simulink model "arm_sim_SMC"  (R2013a)
settings: Solver=ode45  StartTime=0.0  StopTime=100  RelTol=1e-3
undefined symbols (not defined in the file or in its folder): arm_ctrl, drawArm
settings Model: Creator=beard  LastModifiedBy=daqing_yi
settings DataIOCC: SignalLoggingSaveFormat=ModelDataLogs
settings OptimizationCC: ExpressionDepthLimit=2147483647  InitFltsAndDblsToZero=on
settings DebuggingCC: MultiTaskDSMMsg=warning  MultiTaskCondExecSysMsg=none  FcnCallInpInsideContextMsg=UseLocalSettings  StrictBusMsg=None
settings RTWCC: IncludeERTFirstTime=on
settings GRTTargetCC: CombineOutputUpdateFcns=off  GRTInterface=on

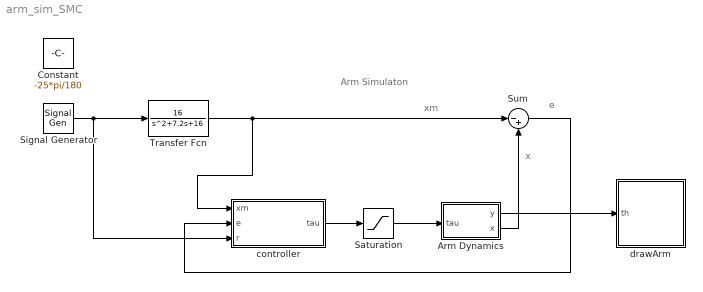
== system arm_sim_SMC ==
  note: x
  note: xm
  note: e
  note: Arm Simulaton
  Arm Dynamics : Subsystem
  Constant : Constant  Value=-25*pi/180
  Saturation : Saturate  UpperLimit=2  LowerLimit=-2
  Signal Generator : SignalGenerator  WaveForm=square  Amplitude=25*pi/180  Frequency=.05
  Sum : Sum  Inputs=|-+
  Transfer Fcn : TransferFcn  Numerator=[16]  Denominator=[1 7.2 16]
  controller : Subsystem
  drawArm : Subsystem
      mask init:
      | % drawing parameters
      | L = 1;
      | w = 0.3;
      mask Display: image(imread('tv.jpg'))
  wires:
  controller/1(tau) -> Saturation/1
  Saturation/1 -> Arm Dynamics/1(tau)
  Arm Dynamics/1(y) -> drawArm/1(th)
  Signal Generator/1 -> controller/3(r), Transfer Fcn/1
  Transfer Fcn/1 -> Sum/1, controller/1(xm)
  Arm Dynamics/2(x) -> Sum/2
  Sum/1 -> controller/2(e)

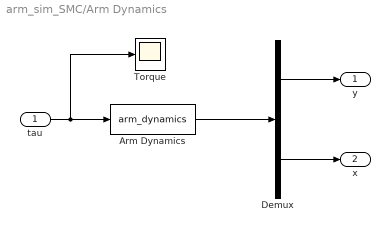
== system arm_sim_SMC/Arm Dynamics ==
  tau : Inport
  Arm Dynamics : S-Function  FunctionName=arm_dynamics  EnableBusSupport=off
  Demux : Demux  Outputs=[1;2]
  Torque : Scope
      settings: TimeRange=100  YMin=-1  YMax=2  SaveName=ScopeData2
  y : Outport
  x : Outport  Port=2
  wires:
  tau/1 -> Arm Dynamics/1, Torque/1
  Arm Dynamics/1 -> Demux/1
  Demux/1 -> y/1
  Demux/2 -> x/1

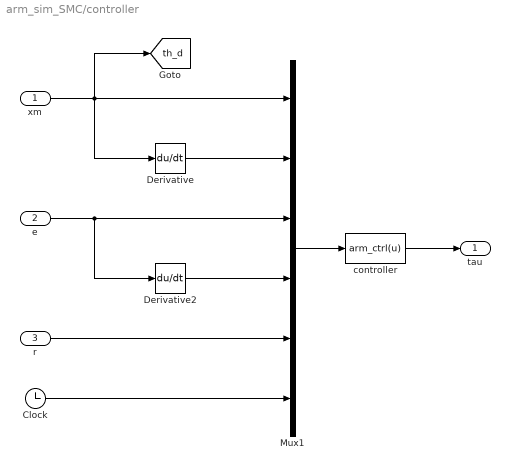
== system arm_sim_SMC/controller ==
  xm : Inport
  e : Inport  Port=2
  r : Inport  Port=3
  Clock : Clock
  Derivative : Derivative
  Derivative2 : Derivative
  Mux1 : Mux  Inputs=6
  controller : MATLABFcn  MATLABFcn=arm_ctrl(u)  OutputDimensions=1  SampleTime=0.01
  tau : Outport
  tag scope: th_d=global
  wires:
  Mux1/1 -> controller/1
  controller/1 -> tau/1
  Clock/1 -> Mux1/6
  xm/1 -> [th_d], Derivative/1, Mux1/1
  Derivative/1 -> Mux1/2
  e/1 -> Mux1/3, Derivative2/1
  Derivative2/1 -> Mux1/4
  r/1 -> Mux1/5

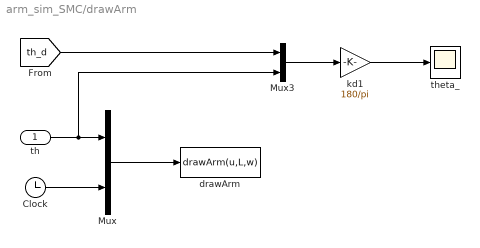
== system arm_sim_SMC/drawArm ==
  th : Inport
  Clock : Clock
  Mux : Mux  Inputs=2
  Mux3 : Mux  Inputs=2
  drawArm : MATLABFcn  MATLABFcn=drawArm(u,L,w)  OutputDimensions=0  SampleTime=0.1
  kd1 : Gain  Gain=180/pi
  theta_ : Scope
      settings: TimeRange=100  YMin=-27.5  YMax=27.5
  wires:
  Mux/1 -> drawArm/1
  th/1 -> Mux3/2, Mux/1
  Clock/1 -> Mux/2
  [th_d] -> Mux3/1
  Mux3/1 -> kd1/1
  kd1/1 -> theta_/1
